simulink model "P4A2"  (R2020a)
settings: Solver=ode45  StartTime=0.0  StopTime=3  RelTol=1e-3
settings Model: Creator=cllau  LastModifiedBy=cllau

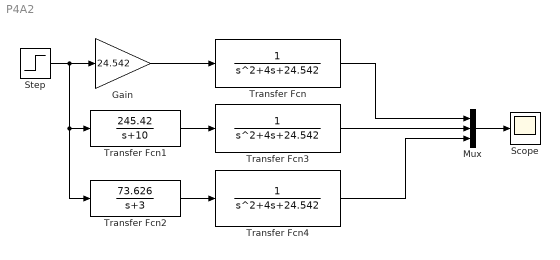
== system P4A2 ==
  Gain : Gain  Gain=24.542
  Mux : Mux  Inputs=3
  Scope : Scope
  Step : Step  Time=0  SampleTime=0
  Transfer Fcn : TransferFcn  Denominator=[1 4 24.542]
  Transfer Fcn1 : TransferFcn  Numerator=[245.42]  Denominator=[1 10]
  Transfer Fcn2 : TransferFcn  Numerator=[73.626]  Denominator=[1 3]
  Transfer Fcn3 : TransferFcn  Denominator=[1 4 24.542]
  Transfer Fcn4 : TransferFcn  Denominator=[1 4 24.542]
  wires:
  Step/1 -> Transfer Fcn2/1, Transfer Fcn1/1, Gain/1
  Transfer Fcn2/1 -> Transfer Fcn4/1
  Transfer Fcn1/1 -> Transfer Fcn3/1
  Gain/1 -> Transfer Fcn/1
  Transfer Fcn/1 -> Mux/1
  Transfer Fcn3/1 -> Mux/2
  Transfer Fcn4/1 -> Mux/3
  Mux/1 -> Scope/1
